simulink model "viptrafficof"  (R2015b)
settings: Solver=FixedStepDiscrete  StartTime=0.0  StopTime=inf  RelTol=1e-3
model workspace (MATLAB code in the model file):
  | line_row =  22;
undefined symbols (not defined in the file or in its folder): gray, Horn, magnitude, Rec, Schunck, SDTV, strel
libraries: visionsinks x4, visiontextngfix x3, visionstatistics x3, visionanalysis x2, visionconversions x1, dspvision x1, vipmisc x1, visionmorphops x1
settings Model: FPTRunName=Active  ExtModeAutoUpdateStatusClock=off  Creator=The MathWorks, Inc.  LastModifiedBy=The MathWorks, Inc.
settings DataIOCC: LimitDataPoints=off  SaveFormat=Array  SaveOutput=off  SignalLogging=off  SaveTime=off  SignalLoggingName=sigsOut
settings OptimizationCC: ExpressionDepthLimit=2147483647  InitFltsAndDblsToZero=on  BufferReusableBoundary=off
settings DebuggingCC: AlgebraicLoopMsg=none  CheckExecutionContextPreStartOutputMsg=on  CheckExecutionContextRuntimeOutputMsg=on  SignalResolutionControl=TryResolveAllWithWarning  MultiTaskDSMMsg=warning  MultiTaskCondExecSysMsg=none  SigSpecEnsureSampleTimeMsg=none  ParameterPrecisionLossMsg=none  FcnCallInpInsideContextMsg=UseLocalSettings  BusObjectLabelMismatch=none  StateNameClashWarn=warning  StrictBusMsg=None
settings HardwareCC: ProdBitPerPointer=32  ProdLargestAtomicFloat=None  ProdIntDivRoundTo=Undefined  ProdEndianess=Unspecified  ProdWordSize=32  ProdHWDeviceType=32-bit Generic  TargetBitPerLong=64  TargetBitPerPointer=64  TargetLongLongMode=on  TargetIntDivRoundTo=Zero  TargetEndianess=LittleEndian  TargetWordSize=64  TargetHWDeviceType=Generic->MATLAB Host Computer  ProdEqTarget=off
settings SFSimCC: SimParseCustomCode=off
settings GRTTargetCC: GeneratePreprocessorConditionals=Disable all  CombineOutputUpdateFcns=off  GRTInterface=on
settings ConfigComp: CovModelRefEnable=Off

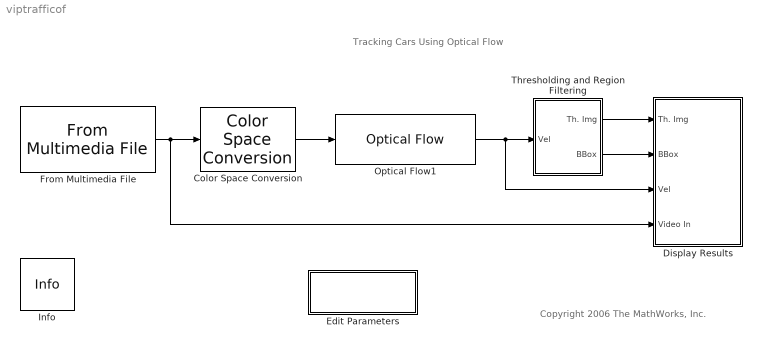
== system viptrafficof ==
  note: Tracking Cars Using Optical Flow
  note: Copyright 2006 The MathWorks, Inc.
  Color Space Conversion : visionconversions/Color Space  Conversion  conversion=Obsolete  conversionActive=R'G'B' to intensity  wp_str=D65  rec=Rec. 601 (SDTV)  sys=1125/60/2:1  imagePorts=One multidimensional signal
  Display Results : Subsystem
  Edit Parameters : Subsystem  mask(Edit Parameters){ofmethod=Horn-Schunck}
      mask prompts: ofmethod "Optical flow estimation method:"
      mask help: Modify model initialization parameters.
      mask init:
      | blk_of= [gcs '/Optical Flow1'];
      | blk_g = [gcs '/Display Results/Optical Flow Lines'];
      | if ofmethod == 1 % HS
      |     set_param(blk_of, 'method', 'Horn-Schunck');
      |     set_param(blk_g,'scaleFactor','20')
      | else
      |     set_param(blk_of, 'method', 'Lucas-Kanade');
      |     set_param(blk_g,'scaleFactor','4')
      | end
      mask TypeOptions ofmethod: Horn-Schunck | Lucas-Kanade
      mask Display: disp('Edit\nParameters')
  From Multimedia File : dspvision/From Multimedia File  inputFilename=viptraffic.avi  loop=on  numPlays=inf  outputStreams=Video only  videoDataType=single  audioDataType=int16  inheritSampleTime=on  userDefinedSampleTime=1/40  noAudioOutput=off  isIntensityVideo=off  fourcc=RGB  colorVideoFormat=One multidimensional signal  outputEOF=off  dataOrg=Column-major  audioFrameSize=1024  computeAudioFrameSize=off  outSamplingMode=Frame based
  Info : vipmisc/Info  SystemSampleTime=-1
  Optical Flow1 : visionanalysis/Optical Flow  method=Horn-Schunck  gradMethod=Difference filter [-1 1]  which2img=Current frame and N-th frame back  N=1  outVelForm=Horizontal and vertical components in complex form  lambda=1  stop_criteria=When maximum number of iterations is reached  maxAllowAbsDiff=eps  maxIter=10  numInports=3  sigmaS=1.5  sigmaW=1  eigTh=0.0039  discardNormalFlow=off  outputCurrentImage=off  prodOutputMode=Binary point scaling  prodOutputWordLength=32  prodOutputFracLength=20  outputMode=Binary point scaling  outputWordLength=32  outputFracLength=20  roundingMode=Nearest  overflowMode=on
  Thresholding and Region Filtering : Subsystem
  wires:
  Thresholding and Region Filtering/2(BBox) -> Display Results/2(BBox)
  Optical Flow1/1 -> Thresholding and Region Filtering/1(Vel), Display Results/3(Vel)
  Color Space Conversion/1 -> Optical Flow1/1
  Thresholding and Region Filtering/1(Th. Img) -> Display Results/1(Th. Img)
  From Multimedia File/1 -> Color Space Conversion/1, Display Results/4(Video In)

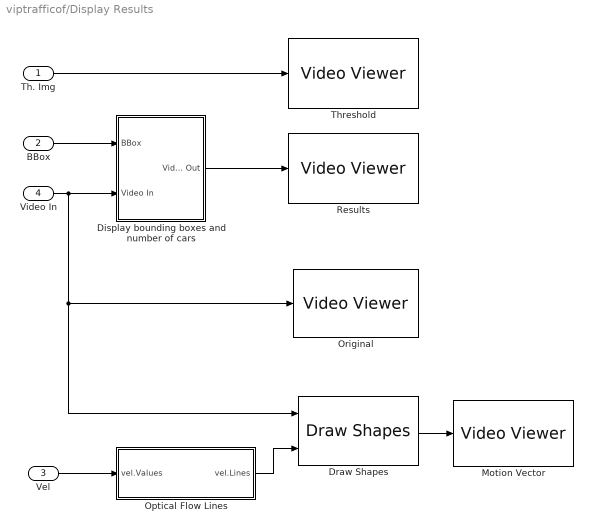
== system viptrafficof/Display Results ==
  Th. Img : Inport
  BBox : Inport  Port=2
  Vel : Inport  Port=3
  Video In : Inport  Port=4
  Display bounding boxes and number of cars : Subsystem
  Draw Shapes : visiontextngfix/Draw Shapes  shape=Lines  fill=off  lineWidth=1  fillClrSource=Specify via dialog  display=User-specified value  intensity=200  color=[255 255 0]  opacity=0.6  viewport=Entire image  antialiasing=off  inType=Obsolete  imagePorts=One multidimensional signal  prodOutputMode=Binary point scaling  prodOutputWordLength=32  prodOutputFracLength=14  memoryMode=Specify word length  memoryWordLength=16  memoryFracLength=15  roundingMode=Floor  overflowMode=off
  Motion Vector : visionsinks/Video Viewer  inputType=Obsolete7b  imagePorts=One multidimensional signal  useColorMap=off  colormapValue=gray(256)  specRange=off  minInputVal=0  maxInputVal=255  FigPos=[335 243 160 142]  AxisZoom=on  trueSizedOnce=on  OpenAtMdlStart=on  DefaultConfigurationName=vipscopes.VideoViewerScopeCfg
  Optical Flow Lines : Subsystem  mask(Optical Flow Lines){scaleFactor=20}
      mask prompts: scaleFactor "Motion vector gain:"
      mask help: Generates the coordinate points of optical flow lines.
      mask Help: Generates the coordinate points of optical flow lines. Look under its mask to see the implementation details.
  Original : visionsinks/Video Viewer  inputType=Obsolete7b  imagePorts=One multidimensional signal  useColorMap=off  colormapValue=gray(256)  specRange=off  minInputVal=0  maxInputVal=255  FigPos=[149 237 160 141]  AxisZoom=on  trueSizedOnce=on  OpenAtMdlStart=on  DefaultConfigurationName=vipscopes.VideoViewerScopeCfg
  Results : visionsinks/Video Viewer  inputType=Obsolete7b  imagePorts=One multidimensional signal  useColorMap=off  colormapValue=gray(256)  specRange=off  minInputVal=0  maxInputVal=255  FigPos=[712 242 163 141]  AxisZoom=on  trueSizedOnce=on  OpenAtMdlStart=on  DefaultConfigurationName=vipscopes.VideoViewerScopeCfg
  Threshold : visionsinks/Video Viewer  inputType=Obsolete7b  imagePorts=One multidimensional signal  useColorMap=off  colormapValue=gray(256)  specRange=off  minInputVal=0  maxInputVal=255  FigPos=[524 242 160 141]  AxisZoom=on  trueSizedOnce=on  OpenAtMdlStart=on  DefaultConfigurationName=vipscopes.VideoViewerScopeCfg
  wires:
  Video In/1 -> Display bounding boxes and number of cars/2(Video In), Original/1, Draw Shapes/1
  Th. Img/1 -> Threshold/1
  BBox/1 -> Display bounding boxes and number of cars/1(BBox)
  Display bounding boxes and number of cars/1(Video Out) -> Results/1
  Draw Shapes/1 -> Motion Vector/1
  Optical Flow Lines/1(vel.Lines) -> Draw Shapes/2
  Vel/1 -> Optical Flow Lines/1(vel.Values)

== system viptrafficof/Edit Parameters ==

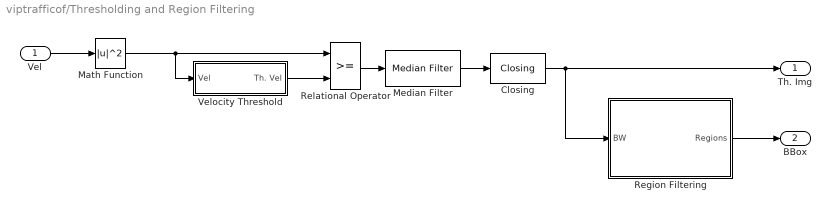
== system viptrafficof/Thresholding and Region Filtering ==
  Vel : Inport
  Closing : visionmorphops/Closing  nhoodsrc=Specify via dialog  strel=strel('line',6,45)
  Math Function : Math  Operator=magnitude^2  SaturateOnIntegerOverflow=on
  Median Filter : visionanalysis/Median Filter  nghbood=[3 3]  outSize=Same as input port I  padType=Constant  padSrc=Specify via dialog  padVal=1  roundingMode=Floor  overflowMode=off
  Region Filtering : Subsystem
  Relational Operator : RelationalOperator  OutDataTypeStr=boolean
  Velocity Threshold : Subsystem
  Th. Img : Outport
  BBox : Outport  Port=2
  wires:
  Closing/1 -> Th. Img/1, Region Filtering/1(BW)
  Median Filter/1 -> Closing/1
  Velocity Threshold/1(Th. Vel) -> Relational Operator/2
  Region Filtering/1(Regions) -> BBox/1
  Vel/1 -> Math Function/1
  Relational Operator/1 -> Median Filter/1
  Math Function/1 -> Velocity Threshold/1(Vel), Relational Operator/1

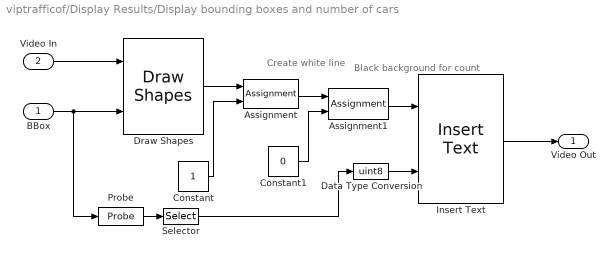
== system viptrafficof/Display Results/Display bounding boxes and number of cars ==
  note: Black background
      | for count
  note: Create white
      | line
  BBox : Inport
  Video In : Inport  Port=2
  Assignment : Assignment  NumberOfDimensions=3  IndexOptions=Index vector (dialog),Assign all,Assign all  Indices=[line_row:line_row+1],[],[]  OutputSizes=1, 1
  Assignment1 : Assignment  NumberOfDimensions=3  IndexOptions=Index vector (dialog),Index vector (dialog),Assign all  Indices=[1:15],[1:30],[]  OutputSizes=1, 1
  Constant : Constant  OutDataTypeStr=single
  Constant1 : Constant  Value=0  OutDataTypeStr=single
  Data Type Conversion : DataTypeConversion  OutDataTypeStr=uint8
  Draw Shapes : visiontextngfix/Draw Shapes  shape=Rectangles  fill=off  lineWidth=1  fillClrSource=Specify via dialog  display=User-specified value  intensity=200  color=[0 1 0]  opacity=0.6  viewport=Entire image  antialiasing=off  inType=Obsolete  imagePorts=One multidimensional signal  prodOutputMode=Binary point scaling  prodOutputWordLength=32  prodOutputFracLength=14  memoryMode=Specify word length  memoryWordLength=16  memoryFracLength=15  roundingMode=Floor  overflowMode=off
  Insert Text : visiontextngfix/Insert Text  inputType=Obsolete  theText='%4d'  getTextLocFrom=Specify via dialog  textLoc=[1 1]  getTextColorFrom=Specify via dialog  textColor=[1 1 1]  getTextIntensityFrom=Specify via dialog  textIntensity=1  getTextOpacityFrom=Specify via dialog  textOpacity=1.0  dummyVar2=0  dummyVar3=0  dummyVar4=0  imagePorts=One multidimensional signal  isInputTransposed=off  fontFace=LucidaTypewriterRegular  dummyVar1=0  blockFontSize=12  antiAliased=on
  Probe : Probe  ProbeWidth=off  ProbeSampleTime=off  ProbeComplexSignal=off  ProbeSignalDimensions=on  ProbeWidthDataType=uint8
  Selector : Selector  NumberOfDimensions=2  InputPortWidth=3  IndexOptions=Index vector (dialog),Index vector (dialog)  Indices=1,1  OutputSizes=99,1
  Video Out : Outport
  wires:
  BBox/1 -> Draw Shapes/2, Probe/1
  Draw Shapes/1 -> Assignment/1
  Assignment/1 -> Assignment1/1
  Constant/1 -> Assignment/2
  Constant1/1 -> Assignment1/2
  Video In/1 -> Draw Shapes/1
  Insert Text/1 -> Video Out/1
  Assignment1/1 -> Insert Text/1
  Probe/1 -> Selector/1
  Selector/1 -> Data Type Conversion/1
  Data Type Conversion/1 -> Insert Text/2

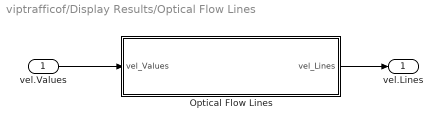
== system viptrafficof/Display Results/Optical Flow Lines ==
  vel.Values : Inport
  Optical Flow Lines : MATLAB Function  TreatAsAtomicUnit=on
  vel.Lines : Outport
  wires:
  Optical Flow Lines/1(vel_Lines) -> vel.Lines/1
  vel.Values/1 -> Optical Flow Lines/1(vel_Values)

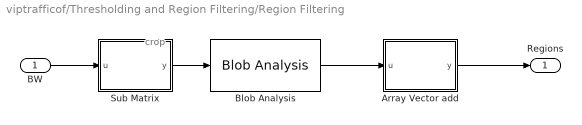
== system viptrafficof/Thresholding and Region Filtering/Region Filtering ==
  note: crop
  BW : Inport
  Array Vector add : MATLAB Function  TreatAsAtomicUnit=on
  Blob Analysis : visionstatistics/Blob Analysis  Tag=vipblks_row_conv  area=off  centroid=off  bBox=on  majorAxis=off  minorAxis=off  angle=off  eccentricity=off  equivDiameterSq=off  extent=off  perimeter=off  maxBlobs=80  warnIfNumBlobsExceeded=on  isCount=off  useMinArea=on  minArea=300  useMaxArea=on  maxArea=3600  excludeBorderBlob=on  outDT=double  isOutVarDim=on  isFill=on  fillValues=-1  conn=8  isLabel=off  outputMode=Binary point scaling  outputWordLength=32  outputFracLength=16  firstCoeffMode=Binary point scaling  firstCoeffWordLength=16  firstCoeffFracLength=14  secondCoeffMode=Binary point scaling  secondCoeffWordLength=32  secondCoeffFracLength=16  accumMode=Binary point scaling  accumWordLength=32  accumFracLength=0  prodOutputMode=Binary point scaling  prodOutputWordLength=32  prodOutputFracLength=16  roundingMode=Floor  overflowMode=off
  Sub Matrix : MATLAB Function  TreatAsAtomicUnit=on
  Regions : Outport
  wires:
  Blob Analysis/1 -> Array Vector add/1(u)
  BW/1 -> Sub Matrix/1(u)
  Array Vector add/1(y) -> Regions/1
  Sub Matrix/1(y) -> Blob Analysis/1

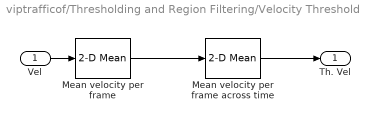
== system viptrafficof/Thresholding and Region Filtering/Velocity Threshold ==
  Vel : Inport
  Mean velocity per frame : visionstatistics/2-D Mean  run=off  reset_popup=None  directionMode=Entire input  dimension=1  treatSBRowAsCol=on  roiEnable=off  roiType=Rectangles  roiPortion=Entire ROI  roiOutput=Individual statistics for each ROI  roiFlag=off  outputDataTypeStr=Inherit: Same as accumulator  outputLastDataTypeStr=Inherit: Same as accumulator  outputMin=[]  outputMax=[]  accumMode=Binary point scaling  accumWordLength=32  accumFracLength=0  accumDataTypeStr=fixdt([],32,0)  accumLastDataTypeStr=fixdt([],32,0)  roundingMode=Floor  overflowMode=off
  Mean velocity per frame across time : visionstatistics/2-D Mean  run=on  reset_popup=None  directionMode=Entire input  dimension=1  treatSBRowAsCol=on  roiEnable=off  roiType=Rectangles  roiPortion=Entire ROI  roiOutput=Individual statistics for each ROI  roiFlag=off  outputDataTypeStr=Inherit: Same as accumulator  outputLastDataTypeStr=Inherit: Same as accumulator  outputMin=[]  outputMax=[]  accumMode=Binary point scaling  accumWordLength=32  accumFracLength=0  accumDataTypeStr=fixdt([],32,0)  accumLastDataTypeStr=fixdt([],32,0)  roundingMode=Floor  overflowMode=off
  Th. Vel : Outport
  wires:
  Mean velocity per frame across time/1 -> Th. Vel/1
  Vel/1 -> Mean velocity per frame/1
  Mean velocity per frame/1 -> Mean velocity per frame across time/1

== matlab function viptrafficof/Display Results/Optical Flow Lines/Optical Flow Lines ==
  data: vel_Values input; vel_Lines output; scaleFactor parameter size=1
function vel_Lines=OpticalFlowLines(vel_Values, scaleFactor) 

% Generates the coordinate points of optical flow lines

persistent first_time;
persistent X;
persistent Y;
persistent RV;
persistent CV;
if isempty(first_time)
    first_time     = 1;
    %% user may change the following three parameters
    borderOffset   = 5;
    decimFactorRow = 5;
    decimFactorCol = 5;    
    %%
    [R C] = size(vel_Values);
    RV = borderOffset:decimFactorRow:(R-borderOffset);   
    CV = borderOffset:decimFactorCol:(C-borderOffset);
    [Y X] = meshgrid(CV,RV);
end

tmp = vel_Values(RV,CV);
tmp = tmp.*scaleFactor;
vel_Lines = [Y(:), X(:), Y(:)+real(tmp(:)), X(:)+imag(tmp(:))];

== matlab function viptrafficof/Thresholding and Region Filtering/Region Filtering/Array Vector add ==
  data: u input size=[80 4] [..320]; y output size=size(u) [..320]; line_row parameter
function y = fcn(u, line_row)
%#codegen
dim=size(u);
repVector = zeros(dim);
repVector=repmat([0 line_row 0 0],dim(1),1); 

y = int32(u+int32(repVector));

== matlab function viptrafficof/Thresholding and Region Filtering/Region Filtering/Sub Matrix ==
  data: u input; y output; line_row parameter
function y = fcn(u, line_row)
%#codegen

l=size(u);

y = u(line_row:l(1),:);
